simulink model "ANN_and_Fuzzy_NCD"  (R2024a)
settings: Solver=ode23  StartTime=0.0  StopTime=200  RelTol=1e-8  EnableMultiTasking=on
model workspace (MAT data in the model file):
  targetSettings3 : object (value not decoded)
values from neighbouring files (symbols this model uses):
  I = in1'    [ann_training.m]
  T = out1'    [ann_training.m]
undefined symbols (not defined in the file or in its folder): B, DL, DQ, m, M, magnitude, rg, W, xb, xg, Xudot, yb, yg, Yvdot, zb, zg, Zwdot
libraries: neural x270, simulink x28, fuzblock x3
(part 12 of 12)

== system ANN_and_Fuzzy_NCD/ ANN x 4  1/Z_1/Layer 3/Delays 1 ==
  "p{3}" : Inport  PortDimensions=10
      mask Display: e = 0.06;c1 = [120 230 180]/255;c2 = ([120 230 180]+0)/(256+128);c3 = ([120 230 180]+128)/(256+128);patch([0 1 1 0],[0 0 1 1],c1);patch([0 1 1 1-e 1-e 0+e],[0 0 1 1-e 0+e 0+e],c2);patch([0 0 1 1-e 0+e 0+e],[0 1 1 1-e 1-e 0+e],c3);plot([0 1 1 0 0],[0 0 1 1 0]);
  mux : Mux  Inputs=1
      mask Display: e = 0.06;c1 = [120 150 230]/255;c2 = ([120 150 230]+0)/383;c3 = ([120 150 230]+128)/383;patch([0 1 1 0],[0 0 1 1],c1);patch([0 1 1 1-e 1-e 0+e],[0 0 1 1-e 0+e 0+e],c2);patch([0 0 1 1-e 0+e 0+e],[0 1 1 1-e 1-e 0+e],c3);plot([0 1 1 0 0],[0 0 1 1 0]);disp('Mux')
  "pd{3,2}" : Outport
      mask Display: e = 0.06;c1 = [120 230 180]/255;c2 = ([120 230 180]+0)/(256+128);c3 = ([120 230 180]+128)/(256+128);patch([0 1 1 0],[0 0 1 1],c1);patch([0 1 1 1-e 1-e 0+e],[0 0 1 1-e 0+e 0+e],c2);patch([0 0 1 1-e 0+e 0+e],[0 1 1 1-e 1-e 0+e],c3);plot([0 1 1 0 0],[0 0 1 1 0]);
  wires:
  "p{3}"/1 -> mux/1
  mux/1 -> "pd{3,2}"/1

== system ANN_and_Fuzzy_NCD/ ANN x 4  1/Z_1/Layer 3/LW{3,2} ==
  "ad{3,2}" : Inport  PortDimensions=10
      mask Display: e = 0.06;c1 = [120 230 180]/255;c2 = ([120 230 180]+0)/(256+128);c3 = ([120 230 180]+128)/(256+128);patch([0 1 1 0],[0 0 1 1],c1);patch([0 1 1 1-e 1-e 0+e],[0 0 1 1-e 0+e 0+e],c2);patch([0 0 1 1-e 0+e 0+e],[0 1 1 1-e 1-e 0+e],c3);plot([0 1 1 0 0],[0 0 1 1 0]);
  "IW{3,2}(1,:)'" : Constant  Value=[-0.0909341668010548165312911805813200771808624267578125;-0.10020375446137445851757519221791881136596202850341796875;0.0004455730783442546382756843659223022768856026232242584228515625;0.1477315993194218413098184328191564418375492095947265625;0.2399540049607259695196859183852211572229862213134765625;0.09675892024341546659993440471225767396390438079833984375;-0.633891886881915667117937118746340274810791015625;-0.412388995987564122014390477488632313907146453857421875;0.1083505744837083006881783830976928584277629852294921875;-0.5541716846373476723641715580015443265438079833984375]
      mask Display: e = 0.06;c1 = [120 150 230]/255;c2 = ([120 150 230]+0)/383;c3 = ([120 150 230]+128)/383;patch([0 1 1 0],[0 0 1 1],c1);patch([0 1 1 1-e 1-e 0+e],[0 0 1 1-e 0+e 0+e],c2);patch([0 0 1 1-e 0+e 0+e],[0 1 1 1-e 1-e 0+e],c3);plot([0 1 1 0 0],[0 0 1 1 0]);disp('weights');
  Mux : Mux  Inputs=1
      mask Display: e = 0.06;c1 = [120 150 230]/255;c2 = ([120 150 230]+0)/383;c3 = ([120 150 230]+128)/383;patch([0 1 1 0],[0 0 1 1],c1);patch([0 1 1 1-e 1-e 0+e],[0 0 1 1-e 0+e 0+e],c2);patch([0 0 1 1-e 0+e 0+e],[0 1 1 1-e 1-e 0+e],c3);plot([0 1 1 0 0],[0 0 1 1 0]);disp('Mux');
  dotprod1 : neural/Weight Functions/dotprod
  "lz{3,2}" : Outport
      mask Display: e = 0.06;c1 = [120 230 180]/255;c2 = ([120 230 180]+0)/(256+128);c3 = ([120 230 180]+128)/(256+128);patch([0 1 1 0],[0 0 1 1],c1);patch([0 1 1 1-e 1-e 0+e],[0 0 1 1-e 0+e 0+e],c2);patch([0 0 1 1-e 0+e 0+e],[0 1 1 1-e 1-e 0+e],c3);plot([0 1 1 0 0],[0 0 1 1 0]);
  wires:
  "IW{3,2}(1,:)'"/1 -> dotprod1/1
  "ad{3,2}"/1 -> dotprod1/2
  dotprod1/1 -> Mux/1
  Mux/1 -> "lz{3,2}"/1

== matlab function ANN_and_Fuzzy_NCD/Euler Transformation 6 DoF1/Environment Impact2/MATLAB Function ==
  data: v_ci output; alpha_c input; beta_c input; V_c input
function v_ci = current_flow(alpha_c,beta_c, V_c)
u_c=V_c*cos(alpha_c)*cos(beta_c);
v_c=V_c*sin(beta_c);
w_c=V_c*sin(alpha_c)*cos(beta_c);
v_ci=[u_c;v_c;w_c;0;0;0];
end

== matlab function ANN_and_Fuzzy_NCD/Euler Transformation 6 DoF/Environment Impact2/MATLAB Function ==
  data: v_ci output; alpha_c input; beta_c input; V_c input
function v_ci = current_flow(alpha_c,beta_c, V_c)
u_c=V_c*cos(alpha_c)*cos(beta_c);
v_c=V_c*sin(beta_c);
w_c=V_c*sin(alpha_c)*cos(beta_c);
v_ci=[u_c;v_c;w_c;0;0;0];
end

== matlab function ANN_and_Fuzzy_NCD/Desired Trajectory2 ==
  settings: updateMethod=DISCRETE
  data: xd input; yd input; zd input; x1 input; y1 input; z1 input; x2 input; y2 input; z2 input
function Trajectory(xd,yd,zd,x1,y1,z1,x2,y2,z2)
persistent Xd Yd Zd X1 Y1 Z1 X2 Y2 Z2 line_handle line_handle1 line_handle2;
if isempty(Xd)
    Xd=[];Yd=[];Zd=[];
    X1=[];Y1=[];Z1=[];
    X2=[];Y2=[];Z2=[];
    figure('Name','ANN and Fuzzy Trajectory');
    hold on;
    xlabel('X Axis');
    ylabel('Y Axis');
    zlabel('Z Axis');
    title('ANN and Fuzzy Trajectory');
    grid on;
    view(45,30);
    line_handle=plot3(NaN,NaN,NaN,'-b');
    line_handle1=plot3(NaN,NaN,NaN,'-b');
    line_handle2=plot3(NaN,NaN,NaN,'-b');
end
Xd=[Xd,xd];
Yd=[Yd,yd];
Zd=[Zd,zd];
X1=[X1,x1];
Y1=[Y1,y1];
Z1=[Z1,z1];
X2=[X2,x2];
Y2=[Y2,y2];
Z2=[Z2,z2];
set(line_handle,'XData',Xd,'YData',Yd,'ZData',Zd);
set(line_handle1,'XData',X1,'YData',Y1,'ZData',Z1,'Color','r');
set(line_handle2,'XData',X2,'YData',Y2,'ZData',Z2,'Color','b');
drawnow;
end
